simulink model "Full_PowerTrain"  (R2024a)
settings: Solver=VariableStepAuto  StartTime=0.0  StopTime=10  RelTol=1e-3
undefined symbols (not defined in the file): Ion, Lithium
libraries: simulink x2, spsBatteryLib x1, spsControlledCurrentSourceLib x1, spsVoltageMeasurementLib x1, sps_lib x1, dspstat3 x1, slpidlib x1
settings Model: Creator=ezeki  LastModifiedBy=ezeki

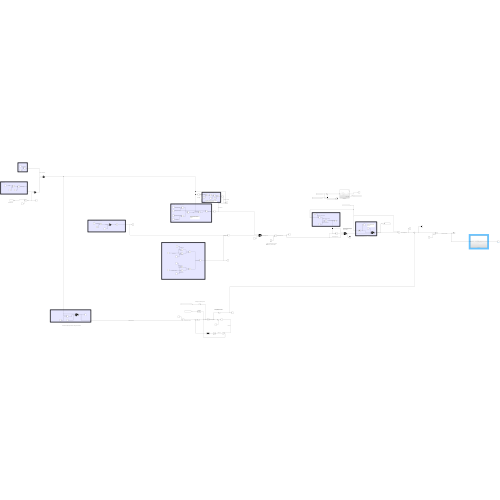
[thumbnail: Simulink's stored preview of the top-level diagram]
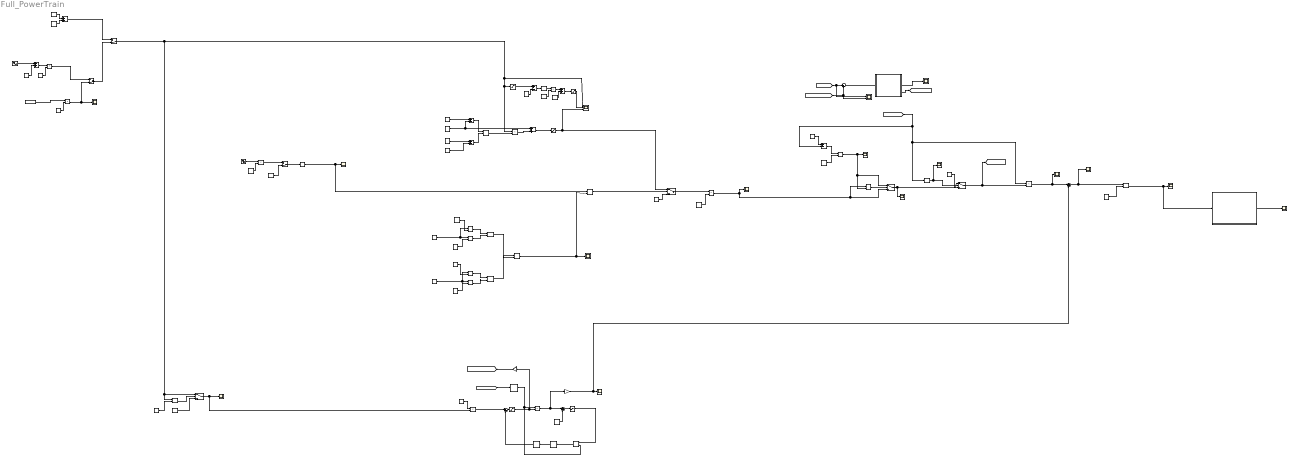
== system Full_PowerTrain ==
  note: This is the threshold for when drive torque is requested, Regen is requested for less then 20%, and throttle is applied for greater then 22%, This gives a 2% deadband
  note: Set sim time to 2154
  note: Inverting as this is a discharge current
  note: Hysterisies Control
  note: Max Charge Current, Regen is scalled 0-100%. Current wants to be 0 -130 amps, therfore scale by 1.3. 600V*130amps = 70kw
  note: If Requested Charge current is greater then permissable charge current then switch to permisable
  note: Throttle ramp (for simulation)
  note: Throttle pedal to regen percentage request
  note: Throttle Input
  note: This function was made in Desmos. Adjusted to meet cross over and start of rise
  note: If Battery Voltage greater then 590 Charge Current is set to zero
  note: Battery Checks
  note: Throttle Mapping to Regen Percentage
  note: throttle output enabled when less then 20% actuation, this will be used for regen
  note: Limiting the input range
  note: Speed Threshold, Regen enabled above 5km/h
  note: Inverting as this is a discharge current, multiple by two to simulate left and right motor controllers
  AND{,1..3} (4 alike) : Logic  IconShape=distinctive  AllPortsSameDT=off  OutDataTypeStr=boolean
  Add{,1..3} (4 alike) : Sum
  Battery Model : Subsystem
  Compare To Constant : simulink/Logic and Bit Operations/Compare To Constant  relop=>  const=5  OutDataTypeStr=boolean
  Constant : Constant  Value=0.5
  Constant1 : Constant  Value=100
  Constant{7,10..11,21,28} (5 alike) : Constant  Value=0
  Constant12 : Constant  Value=6
  Constant13 : Constant  Value=30
  Constant14 : Constant  Value=60
  Constant15 : Constant  Value=0.01
  Constant16 : Constant  Value=50
  Constant17 : Constant  Value=10
  Constant18 : Constant  Value=90
  Constant19 : Constant  Value=5
  Constant2 : Constant  Value=3.6
  Constant20 : Constant  Value=580
  Constant22 : Constant  Value=38000
  Constant23 : Constant  Value=0.75
  Constant24 : Constant
  Constant25 : Constant  Value=100
  Constant27 : Constant  Value=22
  Constant3 : Constant  Value=20
  Constant4 : Constant  Value=10
  Constant5 : Constant  Value=100
  Constant6 : Constant  Value=20
  Constant8 : Constant  Value=20
  Constant9 : Constant  Value=0.25
  Divide{,1..3} (4 alike) : Product  Inputs=*/
  From File : FromFile  FileName=endurancedata.mat  SampleTime=0.01
  Gain : Gain  Gain=-1
  Gain1 : Gain  Gain=-2
  GreaterThan{,1..3} (4 alike) : RelationalOperator  Operator=>  OutDataTypeStr=boolean  RndMeth=Simplest  InputSameDT=off
  IC : InitialCondition  Value=0
  Less Than : RelationalOperator  Operator=<  OutDataTypeStr=boolean  RndMeth=Simplest  InputSameDT=off
  Less Than1 : RelationalOperator  Operator=<  OutDataTypeStr=boolean  RndMeth=Simplest  InputSameDT=off
  Manual Switch : ManualSwitch  CurrentSetting=0
  Manual Switch1 : ManualSwitch  CurrentSetting=0
  Manual Switch2 : ManualSwitch  CurrentSetting=0
  Minus : Sum  Inputs=+-
  Moving Average : dspstat3/Moving Average  Method=Sliding window  ForgettingFactorPort=off  SpecifyWindowLength=on  WindowLength=10  OverlapLength=9  AllowArbitraryInputLength=off  ForgettingFactor=0.9  SimulateUsing=Interpreted execution
  PID Controller : slpidlib/PID Controller  Controller=PID  Form=Parallel  TimeDomain=Continuous-time  UseExternalTs=off  SampleTime=-1  IntegratorMethod=Forward Euler  FilterMethod=Forward Euler  ControllerParametersSource=internal  P=0.000129604741819679  I=2.74416284727287  UseKiTs=off  D=0  UseExternalDerivativeSource=off  N=100  UseFilter=on  TunerSelectOption=Transfer Function Based (PID Tuner App)  InitialConditionSource=internal  InitialConditionForIntegrator=10  InitialConditionForFilter=0  DifferentiatorICPrevScaledInput=0  ExternalReset=none  TrackingMode=off  Kt=1  LimitOutput=off  SatLimitsSource=internal  UpperSaturationLimit=inf  LowerSaturationLimit=-inf  LinearizeAsGain=on  AntiWindupMode=none  Kb=1  LimitIntegrator=off  UpperIntegratorSaturationLimit=inf  LowerIntegratorSaturationLimit=-inf  POutMin=[]  POutMax=[]  IOutMin=[]  IOutMax=[]  DOutMin=[]  DOutMax=[]  NOutMin=[]  NOutMax=[]  SumOutMin=[]  SumOutMax=[]  SaturationOutMin=[]  SaturationOutMax=[]  PParamMin=[]  PParamMax=[]  IParamMin=[]  IParamMax=[]  DParamMin=[]  DParamMax=[]  NParamMin=[]  NParamMax=[]  KbParamMin=[]  KbParamMax=[]  KtParamMin=[]  KtParamMax=[]  KbOutMin=[]  KbOutMax=[]  KtOutMin=[]  KtOutMax=[]  IntegratorOutMin=[]  IntegratorOutMax=[]  FilterOutMin=[]  FilterOutMax=[]  SumI1OutMin=[]  SumI1OutMax=[]  SumI2OutMin=[]  SumI2OutMax=[]  SumI3OutMin=[]  SumI3OutMax=[]  SumI4OutMin=[]  SumI4OutMax=[]  SumDOutMin=[]  SumDOutMax=[]  DifferentiatorOutMin=[]  DifferentiatorOutMax=[]  FilterDiffOutCoefMin=[]  FilterDiffOutCoefMax=[]  ReciprocalOutMin=[]  ReciprocalOutMax=[]  SumDenOutMin=[]  SumDenOutMax=[]  SumNumOutMin=[]  SumNumOutMax=[]  DivideOutMin=[]  DivideOutMax=[]  UdiffTsProdOutMin=[]  UdiffTsProdOutMax=[]  NTsProdOutMin=[]  NTsProdOutMax=[]  UintegralTsProdOutMin=[]  UintegralTsProdOutMax=[]  UngainTsProdOutMin=[]  UngainTsProdOutMax=[]  ClampingZeroOutDataTypeStr=Inherit: Inherit via back propagation  ClampingZeroOutMin=[]  ClampingZeroOutMax=[]  FilterDenConstantOutDataTypeStr=Inherit: Inherit via back propagation  FilterDenConstantOutMin=[]  FilterDenConstantOutMax=[]  PCopyOutDataTypeStr=Inherit: Inherit via back propagation  PCopyOutMin=[]  PCopyOutMax=[]  NCopyOutDataTypeStr=Inherit: Inherit via back propagation  NCopyOutMin=[]  NCopyOutMax=[]  IntegratorContinuousStateAttributes=''  IntegratorStateMustResolveToSignalObject=off  IntegratorRTWStateStorageClass=Auto  FilterContinuousStateAttributes=''  FilterStateMustResolveToSignalObject=off  FilterRTWStateStorageClass=Auto  ParallelPVariant=InternalParameters  IdealPVariant=Disabled  IVariant=InternalParameters  DVariant=InternalParameters  IntegratorVariant=Continuous  SatVariant=Disabled  AWVariant=Passthrough  PCopyVariant=Disabled  TRVariant=Disabled  FdbkBlocksVariant=Forward  IdealPFdbkVariant=Disabled  SatFdbkVariant=Disabled  DerivativeFilterVariant=ContFilter  NVariant=InternalParameters  NCopyVariant=Disabled  FilterICVariant=InternalICsFilter  IntegratorICVariant=InternalICs  ExternalResetVariant=Disabled  TRSumVariant=Passthrough  SumFdbkVariant=Disabled  SumVariant=Sum_PID  TsampFilterVariant=InternalTs  TsampNgainVariant=Passthrough  TsampIntegralVariant=Disabled_SignalSpec  ExternalSaturationOutDataTypeStr=Inherit: Same as second input  DerivativeSourceVariant=ErrorSignal
  Product{,1..8} (9 alike) : Product
  Ramp : simulink/Sources/Ramp  slope=-2  start=0  InitialOutput=0
  Relay : Relay  OnSwitchValue=590  OffSwitchValue=585  OnOutputValue=0  OffOutputValue=1
  Saturation : Saturate  UpperLimit=100  LowerLimit=0
  Saturation1 : Saturate  UpperLimit=100  LowerLimit=0
  Saturation2 : Saturate  UpperLimit=20  LowerLimit=0
  Saturation3 : Saturate  UpperLimit=inf  LowerLimit=0
  Saturation5 : Saturate  UpperLimit=inf  LowerLimit=0
  Scale : Constant  Value=1.3
  Scope{,1,3..9,11..14,17} (14 alike) : Scope
  Scope10 : Scope  NumInputPorts=2
  Scope2 : Scope  NumInputPorts=3
  Sine Wave : Sin  Amplitude=0.5  SampleTime=0
  Sine Wave1 : Sin  SampleTime=0
  Square : Math  Operator=square
  Subsystem : Subsystem
  Subtract : Sum  Inputs=+-
  Subtract1 : Sum  Inputs=+-
  Subtract2 : Sum  Inputs=+-
  Sum : Sum  Inputs=|+-
  Sum1 : Sum  Inputs=|+-
  Sum2 : Sum  Inputs=|++
  Sum3 : Sum  Inputs=|++
  Switch : Switch  Criteria=u2 > Threshold  SaturateOnIntegerOverflow=off  InputSameDT=off
  Switch1 : Switch  Criteria=u2 > Threshold  SaturateOnIntegerOverflow=off  InputSameDT=off
  Switch2 : Switch  Criteria=u2 > Threshold  Threshold=0.5  SaturateOnIntegerOverflow=off  InputSameDT=off
  Switch3 : Switch  Criteria=u2 > Threshold  SaturateOnIntegerOverflow=off  InputSameDT=off
  wires:
  Scale/1 -> Product4/2
  Product4/1 -> Scope/1, Switch1/3, GreaterThan2/1  "Requested Charge Current"
  Relay/1 -> Switch2/2, Scope7/1
  GreaterThan2/1 -> Switch1/2
  Constant20/1 -> Minus/1  "Max Battery Voltage using Regen"
  Minus/1 -> Divide/1  "Voltage Threshold to overcharge"
  Constant21/1 -> Switch2/3
  Switch2/1 -> Product7/2, [Requested_Current]  "Charge Current"
  Constant15/1 -> Divide/2  "Battery Internal Resistance"
  Switch/1 -> Product4/1  "Requested Charge Current"
  [Battery_Voltage] -> Minus/2, Product7/1, Relay/1
  Divide/1 -> GreaterThan2/2, Switch1/1, Scope9/1  "Maximum Permissable Charge Current"
  Constant4/1 -> Subtract/1  "Min Regen Percentage"
  AND2/1 -> AND3/2
  AND1/1 -> AND3/1
  Constant18/1 -> Less Than1/2  "Max Battery SOC"
  Less Than1/1 -> AND2/2
  Less Than/1 -> AND1/2
  Product2/1 -> Add3/2
  GreaterThan/1 -> AND1/1
  AND3/1 -> Scope3/1, AND/2  "Battery Logic"
  GreaterThan1/1 -> AND2/1
  Constant12/1 -> Manual Switch1/2
  Subtract2/1 -> Square/1
  Add1/1 -> Manual Switch/1  "Throttle Pedal Simulated"
  Constant13/1 -> GreaterThan/1, Less Than/1  "Battery Temp"
  Manual Switch1/1 -> Compare To Constant/1
  Sine Wave/1 -> Add/1  "Throttle"
  Product3/1 -> Add2/1
  Constant17/1 -> GreaterThan/2  "Min Battery Temp"
  Constant11/1 -> Switch/3
  Manual Switch/1 -> Switch3/1, GreaterThan3/1, Product2/1, Saturation2/1, Scope2/1  "Throttle Pedal"
  AND/1 -> Switch/2
  Constant14/1 -> GreaterThan1/1, Less Than1/1  "Battery State of Charge"
  Constant5/1 -> Subtract/2, Add3/1  "Max Regen Percentage"
  Saturation2/1 -> Subtract2/1  "Exponential Throttle Map"
  Ramp/1 -> Add1/1  "Throttle Pedal"
  Divide1/1 -> Product2/2  "Slope"
  Constant10/1 -> Add2/2
  Constant3/1 -> Subtract2/2
  Constant8/1 -> Add1/2
  Saturation/1 -> Switch/1, Scope2/3  "Linear Regen Map"
  Add3/1 -> Saturation/1  "Regen Request"
  Subtract/1 -> Divide1/1
  Subtract1/1 -> Divide1/2
  Square/1 -> Product3/1
  Add2/1 -> Saturation1/1
  Saturation1/1 -> Scope2/2  "Exponential Throttle Map"
  Constant9/1 -> Product3/2
  Constant/1 -> Add/2  "Offset"
  Constant19/1 -> GreaterThan1/2  "Min Battery SOC"
  Add/1 -> Product/1
  Product/1 -> Manual Switch2/1  "Throttle Percentage"
  Constant1/1 -> Product/2
  Compare To Constant/1 -> AND/1, Scope1/1
  Product1/1 -> Manual Switch1/1  "Speed (km/h)"
  Sine Wave1/1 -> Product1/1  "Speed (m/s)"
  Constant2/1 -> Product1/2
  Constant7/1 -> Subtract1/2  "Intial distance"
  Constant16/1 -> Less Than/2  "Max Battery temp"
  Constant6/1 -> Subtract1/1  "Minimum Throttle Percentage"
  GreaterThan3/1 -> Switch3/2
  Constant27/1 -> GreaterThan3/2
  Constant28/1 -> Switch3/3
  Switch3/1 -> Product6/2, Scope14/1  "Throttle Percentage > 20"
  Product6/1 -> Sum/1  "Current Request (0-75amps)"
  PID Controller/1 -> IC/1
  Sum/1 -> Saturation5/1
  Saturation3/1 -> Divide2/1  "Power Error"
  Constant22/1 -> Sum1/2
  Product5/1 -> Sum1/1, Gain1/1  "Requested Discharge Power"
  Moving Average/1 -> Divide2/2, Product5/1
  IC/1 -> Sum/2
  Sum1/1 -> Saturation3/1
  Divide2/1 -> PID Controller/1  "Current Error"
  Gain/1 -> [Requested_Current_Discharge]
  Saturation5/1 -> Gain/1, Product5/2
  Constant23/1 -> Product6/1
  [Requested_Current] -> Scope10/1, Sum2/1
  Battery Model/3(Batter Voltage) -> [Battery_Voltage]
  [Battery_Voltage] -> Moving Average/1
  Sum2/1 -> Battery Model/1(s)
  [Requested_Current_Discharge] -> Sum2/2, Scope10/2
  Battery Model/2(Out2) -> Scope4/1
  Product7/1 -> Scope13/1, Sum3/1  "Requested Charge Power"
  Sum3/1 -> Scope11/1, Divide3/1
  Constant24/1 -> Divide3/2  "Motor RPM"
  Divide3/1 -> Subsystem/1(Torque Request), Scope6/1  "Torque Request to Motors"
  Gain1/1 -> Sum3/2, Scope5/1
  Product8/1 -> Scope12/1, Manual Switch2/2  "Throttle"
  Manual Switch2/1 -> Manual Switch/2
  Constant25/1 -> Product8/2
  From File/1 -> Product8/1  "Throttle"
  Switch1/1 -> Switch2/1, Scope8/1
  Subsystem/1(Over Current Protected Torque Request to Inverters) -> Scope17/1

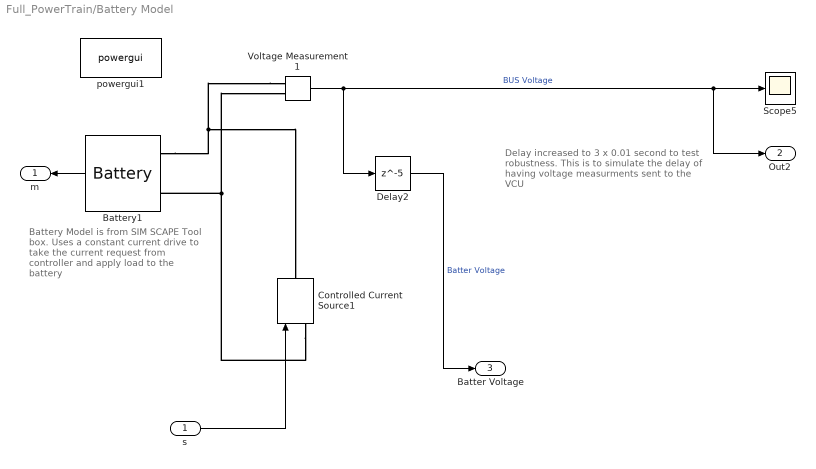
== system Full_PowerTrain/Battery Model ==
  note: Delay increased to 3 x 0.01 second to test robustness. This is to simulate the delay of having voltage measurments sent to the VCU
  note: Battery Model is from SIM SCAPE Tool box. Uses a constant current drive to take the current request from controller and apply load to the battery
  s : Inport
  Battery1 : spsBatteryLib/Battery  BatType=Lithium-Ion  ShowTempParam=off  ThermalPreset=no  ShowAgeParam=off  NomV=532.8  NomQ=1152  SOC=85  Batt_Tr=5  PresetModel=on  MaxQ=1152  MinV=399.6  FullV=620.1723  Dis_rate=500.8696  R=0.004625  Normal_OP=1041.8087  expZone="[575.6296      56.59826]"  current=[6.5 13 32.5]  Units=Time  Tci=20  NomT=20  T2=-30  MaxQ2=4.8  FullV2=7.1  Normal_OP2=5.655  expZone2="[6.58           1]"  Rca=0.6  ti=2000  Dp=0  Neq0=0  Tsim=1e6  Ta1=25  Qeol=5.4*0.9  Reol=0.013333*1.2  Char_age=[2.3478, 3]  Dis_age=[2.3478, 10]  N1=1500  N2=10500  N3=1000  N4=1400  Ta2=45  N5=950
  Controlled Current Source1 : spsControlledCurrentSourceLib/Controlled Current Source  Initialize=on  Source_Type=AC  Amplitude=0  Phase=0  Frequency=0  Measurements=None
  Delay2 : Delay  DelayLength=5  InitialCondition=580
  Scope5 : Scope
  Voltage Measurement1 : spsVoltageMeasurementLib/Voltage Measurement  PhasorSimulation=off  OutputType=Complex  PSBequivalent=0
  powergui1 : sps_lib/powergui  Priority=1  SimulationMode=Discrete  SampleTime=0.01  frequency=60  Iterations=50  frequencyindice=0  Pbase=100e6  ErrMax=1e-4  UnitsV=kV  UnitsW=MW  buscounter=0  FunctionMessages=off  echomessages=off  EnableUseOfTLC=off  CurrentSourceSwitches=off  DisableSnubberDevices=off  DisableRonSwitches=off  DisableVfSwitches=off  DisplayEquations=off  AutomaticDiscreteSolvers=off  SolverType=Tustin/Backward Euler (TBE)  Interpol=off  ExternalGateDelay=off  methode=off  Ts=100  x0status=blocks  SPID=on  SwTol=0  HookPort=off  NonlinearTolerance=1e-4  nMaxIteration=100  ContinueOnMaxIteration=off  RestoreLinks=warning  ResistiveCurrentMeasurement=off  Frange=[0:2:500]  Ylog=off  Xlog=on  ShowGrid=off  save=off  variable=ZData  structure=0  ZoomFFT=off  StartTime=0.0  cycles=1  DisplayStyle=1  fundamental=60  FreqAxis=off  MaxFrequency=1000  frequencyindicesteady=1  RmsSteady=1  display=off
  m : Outport
  Out2 : Outport  Port=2
  Batter Voltage : Outport  Port=3
  wires:
  Voltage Measurement1/1 -> Delay2/1, Out2/1, Scope5/1  "BUS Voltage"
  s/1 -> Controlled Current Source1/1
  Delay2/1 -> Batter Voltage/1  "Batter Voltage"
  Battery1/1 -> m/1
  connections:
  Voltage Measurement1/LConn1 -- Controlled Current Source1/RConn1 -- Battery1/LConn1
  Battery1/LConn2 -- Voltage Measurement1/LConn2 -- Controlled Current Source1/LConn1

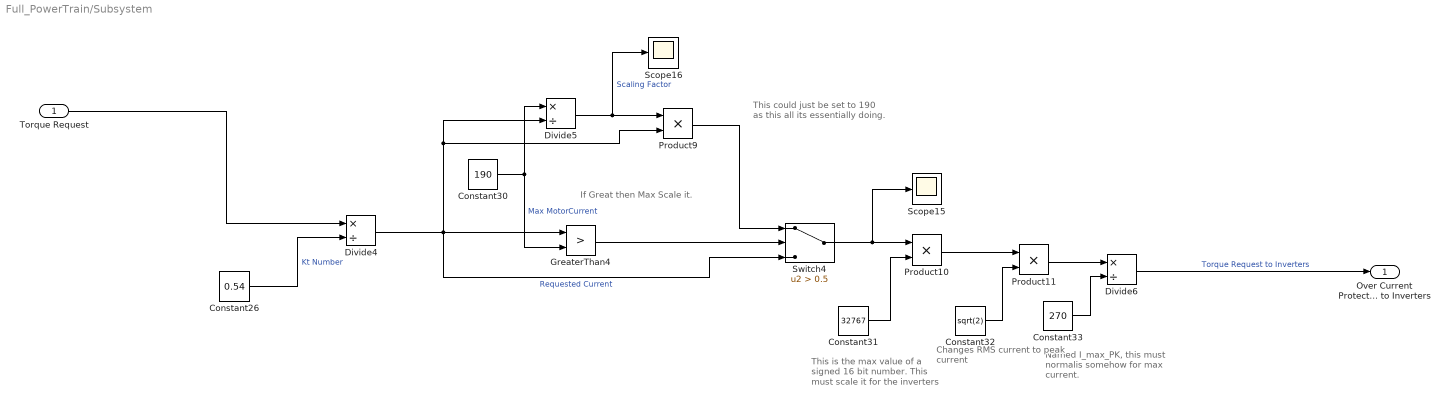
== system Full_PowerTrain/Subsystem ==
  note: This could just be set to 190 as this all its essentially doing.
  note: Named I_max_PK, this must normalis somehow for max current.
  note: Changes RMS current to peak current
  note: This is the max value of a signed 16 bit number. This must scale it for the inverters
  note: If Great then Max Scale it.
  Torque Request : Inport
  Constant26 : Constant  Value=0.54
  Constant30 : Constant  Value=190
  Constant31 : Constant  Value=32767
  Constant32 : Constant  Value=sqrt(2)
  Constant33 : Constant  Value=270
  Divide4 : Product  Inputs=*/
  Divide5 : Product  Inputs=*/
  Divide6 : Product  Inputs=*/
  GreaterThan4 : RelationalOperator  Operator=>  OutDataTypeStr=boolean  RndMeth=Simplest  InputSameDT=off
  Product10 : Product
  Product11 : Product
  Product9 : Product
  Scope15 : Scope
  Scope16 : Scope
  Switch4 : Switch  Criteria=u2 > Threshold  Threshold=0.5  SaturateOnIntegerOverflow=off  InputSameDT=off
  Over Current Protected Torque Request to Inverters : Outport
  wires:
  Constant31/1 -> Product10/2
  Product10/1 -> Product11/1
  Constant33/1 -> Divide6/2
  GreaterThan4/1 -> Switch4/2
  Divide5/1 -> Scope16/1, Product9/1  "Scaling Factor"
  Constant30/1 -> Divide5/1, GreaterThan4/2  "Max MotorCurrent"
  Product9/1 -> Switch4/1
  Divide4/1 -> Product9/2, Divide5/2, Switch4/3, GreaterThan4/1  "Requested Current"
  Constant26/1 -> Divide4/2  "Kt Number"
  Switch4/1 -> Product10/1, Scope15/1
  Constant32/1 -> Product11/2
  Product11/1 -> Divide6/1
  Torque Request/1 -> Divide4/1
  Divide6/1 -> Over Current Protected Torque Request to Inverters/1  "Torque Request to Inverters"
